simulink model "SL_0"  (R2025a)
settings: Solver=VariableStepAuto  StartTime=0.0  StopTime=10e-3  MaxStep=1e-3/50  RelTol=1e-3
settings Model: Creator=Szalay  LastModifiedBy=Szalay

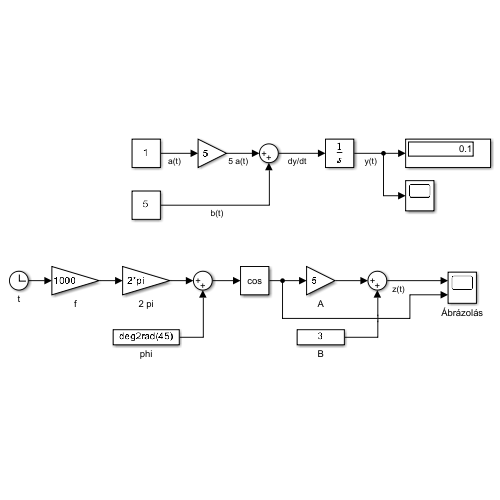
[thumbnail: Simulink's stored preview of the top-level diagram]
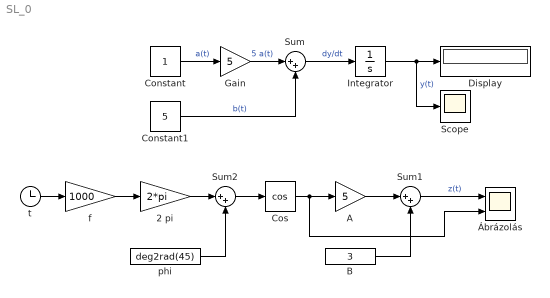
== system SL_0 ==
  2 pi : Gain  Gain=2*pi
  A : Gain  Gain=5
  B : Constant  Value=3
  Constant : Constant
  Constant1 : Constant  Value=5
  Cos : Trigonometry  Operator=cos
  Display : Display
  Gain : Gain  Gain=5
  Integrator : Integrator
  Scope : Scope
      settings: ActiveDisplayYMinimum=-1  ActiveDisplayYMaximum=1
  Sum : Sum  Inputs=|++
  Sum1 : Sum  Inputs=|++
  Sum2 : Sum  Inputs=|++
  f : Gain  Gain=1000
  phi : Constant  Value=deg2rad(45)
  t : Clock
  Ábrázolás : Scope  NumInputPorts=2
      settings: ActiveDisplayYMinimum=-3.246916002285881  ActiveDisplayYMaximum=9.2469160022859018
  wires:
  Constant/1 -> Gain/1  "a(t)"
  Constant1/1 -> Sum/2  "b(t)"
  Sum/1 -> Integrator/1  "dy/dt"
  Gain/1 -> Sum/1  "5 a(t)"
  Integrator/1 -> Scope/1, Display/1  "y(t)"
  A/1 -> Sum1/1
  B/1 -> Sum1/2
  Cos/1 -> Ábrázolás/2, A/1
  Sum2/1 -> Cos/1
  phi/1 -> Sum2/2
  2 pi/1 -> Sum2/1
  f/1 -> 2 pi/1
  t/1 -> f/1
  Sum1/1 -> Ábrázolás/1  "z(t)"
